simulink model "tri1"  (R2016b)
settings: Solver=VariableStepAuto  StartTime=0.0  StopTime=20  RelTol=1e-3
settings Model: Creator=Admin  LastModifiedBy=Admin

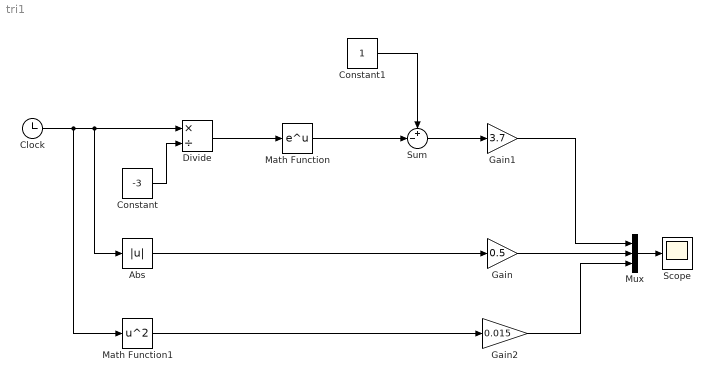
== system tri1 ==
  Abs : Abs
  Clock : Clock
  Constant : Constant  Value=-3
  Constant1 : Constant
  Divide : Product  Inputs=*/
  Gain : Gain  Gain=0.5
  Gain1 : Gain  Gain=3.7
  Gain2 : Gain  Gain=0.015
  Math Function : Math  SaturateOnIntegerOverflow=on
  Math Function1 : Math  Operator=square  SaturateOnIntegerOverflow=on
  Mux : Mux  Inputs=3
  Scope : Scope
  Sum : Sum  Inputs=+-|
  wires:
  Clock/1 -> Math Function1/1, Abs/1, Divide/1
  Constant/1 -> Divide/2
  Divide/1 -> Math Function/1
  Math Function/1 -> Sum/2
  Constant1/1 -> Sum/1
  Sum/1 -> Gain1/1
  Abs/1 -> Gain/1
  Math Function1/1 -> Gain2/1
  Gain1/1 -> Mux/1
  Gain/1 -> Mux/2
  Gain2/1 -> Mux/3
  Mux/1 -> Scope/1
